simulink model "SF007A_SysFricLrng"  (R2013b)
settings: Solver=FixedStepDiscrete  SolverMode=SingleTasking  StartTime=0.0  StopTime=1  FixedStep=0.002  RelTol=1e-3
PostLoadFcn:
  | , if any(exist('dsrtsu_mdlpostloadfcn', 'file') == [2, 3, 6]), try dsrtsu_mdlpostloadfcn('Execute', bdroot); catch fprintf('Error in PostLoadFcn (dsrtsu_mdlpostloadfcn) for model "%s":\n %s\n', bdroot, lasterr); end, end,
values from neighbouring files (symbols this model uses):
  ARCHGLBPRM_100MILLISEC_SEC_F32 = DataDict.Constant    [SF007A_SysFricLrng_DataDict.m]
  ARCHGLBPRM_10MILLISEC_SEC_F32 = DataDict.Constant    [SF007A_SysFricLrng_DataDict.m]
  ARCHGLBPRM_180OVERPI_ULS_F32 = DataDict.Constant    [SF007A_SysFricLrng_DataDict.m]
  CONV100MICROSECTOSEC_ULS_F32 = DataDict.Constant    [SF007A_SysFricLrng_DataDict.m]
  FLTINJ_SYSFRICLRNG_SYSFRICOFFS = DataDict.Constant    [SF007A_SysFricLrng_DataDict.m]
  FricLrngData = DataDict.NVM    [SF007A_SysFricLrng_DataDict.m]
  HWPTNUM_CNT_U08 = DataDict.Constant    [SF007A_SysFricLrng_DataDict.m]
  HWPTNUMSUB1_CNT_U08 = DataDict.Constant    [SF007A_SysFricLrng_DataDict.m]
  HWVELDECDIR_ULS_U08 = DataDict.Constant    [SF007A_SysFricLrng_DataDict.m]
  HWVELINCDIR_ULS_U08 = DataDict.Constant    [SF007A_SysFricLrng_DataDict.m]
  IDXCALCNSCAGFAC_ULS_U08 = DataDict.Constant    [SF007A_SysFricLrng_DataDict.m]
  IDXSELN1_ULS_U08 = DataDict.Constant    [SF007A_SysFricLrng_DataDict.m]
  IDXSELN2_ULS_U08 = DataDict.Constant    [SF007A_SysFricLrng_DataDict.m]
  IDXSELN3_ULS_U08 = DataDict.Constant    [SF007A_SysFricLrng_DataDict.m]
  LRNGENASCAFAC_MILLISEC_U32 = DataDict.Constant    [SF007A_SysFricLrng_DataDict.m]
  SCAGFACQUARTER_CNT_F32 = DataDict.Constant    [SF007A_SysFricLrng_DataDict.m]
  SCAGFACTEN_CNT_U16 = DataDict.Constant    [SF007A_SysFricLrng_DataDict.m]
  SCAGFACVEHLATA_MTRPERSECSQD_F32 = DataDict.Constant    [SF007A_SysFricLrng_DataDict.m]
  SECIDXSELN_ULS_U08 = DataDict.Constant    [SF007A_SysFricLrng_DataDict.m]
  SysFricLrngBasLineEolFric = DataDict.Calibration    [SF007A_SysFricLrng_DataDict.m]
  SysFricLrngBasLineFric = DataDict.Calibration    [SF007A_SysFricLrng_DataDict.m]
  SysFricLrngBasLineHys = DataDict.Calibration    [SF007A_SysFricLrng_DataDict.m]
  SysFricLrngBasLineRngCntr = DataDict.Calibration    [SF007A_SysFricLrng_DataDict.m]
  SysFricLrngEolFricDifScagFac = DataDict.Calibration    [SF007A_SysFricLrng_DataDict.m]
  SysFricLrngFricChgWght = DataDict.Calibration    [SF007A_SysFricLrng_DataDict.m]
  SysFricLrngFricDiagcThd = DataDict.Calibration    [SF007A_SysFricLrng_DataDict.m]
  SysFricLrngFricDiagcTiThd = DataDict.Calibration    [SF007A_SysFricLrng_DataDict.m]
  SysFricLrngFricHysHwAgPt = DataDict.Calibration    [SF007A_SysFricLrng_DataDict.m]
  SysFricLrngGain = DataDict.Calibration    [SF007A_SysFricLrng_DataDict.m]
  SysFricLrngHwPosnAuthyThd = DataDict.Calibration    [SF007A_SysFricLrng_DataDict.m]
  SysFricLrngHwVelConstrLim = DataDict.Calibration    [SF007A_SysFricLrng_DataDict.m]
  SysFricLrngHwVelHiLim = DataDict.Calibration    [SF007A_SysFricLrng_DataDict.m]
  SysFricLrngHwVelLoLim = DataDict.Calibration    [SF007A_SysFricLrng_DataDict.m]
  SysFricLrngIgnCycFricChgLim = DataDict.Calibration    [SF007A_SysFricLrng_DataDict.m]
  SysFricLrngLatAHiLim = DataDict.Calibration    [SF007A_SysFricLrng_DataDict.m]
  SysFricLrngLatALoLim = DataDict.Calibration    [SF007A_SysFricLrng_DataDict.m]
  SysFricLrngMaskVehSpd = DataDict.Calibration    [SF007A_SysFricLrng_DataDict.m]
  SysFricLrngRngCntrThd = DataDict.Calibration    [SF007A_SysFricLrng_DataDict.m]
  SysFricLrngThd = DataDict.Calibration    [SF007A_SysFricLrng_DataDict.m]
  SysFricLrngTHiLim = DataDict.Calibration    [SF007A_SysFricLrng_DataDict.m]
  SysFricLrngTLoLim = DataDict.Calibration    [SF007A_SysFricLrng_DataDict.m]
  SysFricLrngVehSpd = DataDict.Calibration    [SF007A_SysFricLrng_DataDict.m]
  SYSFRICOFFSLIM_HWNWTMTR_F32 = DataDict.Constant    [SF007A_SysFricLrng_DataDict.m]
  VEHSPDPTNUM1_ULS_U08 = DataDict.Constant    [SF007A_SysFricLrng_DataDict.m]
  VEHSPDPTNUM2_ULS_U08 = DataDict.Constant    [SF007A_SysFricLrng_DataDict.m]
undefined symbols (not defined in the file or in its folder): NtcNr1, NtcSts1, SysFricLrngOperMod1
libraries: Fil x19, simulink x17, NxtrLim x10, NxtrAbslt x3, NxtrNvM x2, FixdToFloat x2, FloatToFixd x1, LnrIntrpn x1
(part 3 of 7)

== system SF007A_SysFricLrng/SysFricLrng/SysFricLrngPer1/RunningAndCalibrationModes/CalMode ==
  Action Port : ActionPort  ActionType=then
  Constant1 : Constant  Value=0  OutDataTypeStr=single
      settings: AttributesFormatString=%<OutDataTypeStr>
  Constant2 : Constant  Value=0  OutDataTypeStr=single
      settings: AttributesFormatString=%<OutDataTypeStr>
  CopyRight2 : Subsystem  Description=|  mask(Copyright Information){none=on}
      | Copyright info block.                                               
      |                                                                     
      | Place copyright information at the top of every subsystem in design.
      mask prompts: none "No parameters"
      mask help: Place copyright information at the top of every subsystem in design.
      mask Display:
      | NxtrConf = 'Nexteer Confidential';
      | 
      | sys = bdroot; %handle for the current model ("system")
      | first = get_param(sys,'Created');
      | first = first(end-3:end);  %year is last four digits
      | 
      | last = get_param(sys,'LastModifiedDate');
      | if isempty(last)
      |     last = datestr(now,'yyyy');
      | else
      |     last = last(end-3:end);
      | end
      | 
      | if strcmp(first,last)
      |     fprintf('%s -- Copyright %s Nexteer',NxtrConf,first)
      | else
      |     fprintf('%s -- %s%s- %s Nexteer',NxtrConf,char(169),first,last)
      | end
  Data Store Read3 : DataStoreRead  DataStoreName=SatnAvrgFric
  Data Store Write : DataStoreWrite  DataStoreName=VehBasLineFric
  Data Store Write1 : DataStoreWrite  DataStoreName=FricChgLpFil  DataStoreElements=FricChgLpFil.FilSt
  FricOffs : Outport  InitialOutput=[0]
  wires:
  Data Store Read3/1 -> Data Store Write/1
  Constant1/1 -> FricOffs/1
  Constant2/1 -> Data Store Write1/1

== system SF007A_SysFricLrng/SysFricLrng/SysFricLrngPer1/RunningAndCalibrationModes/CopyRight2 ==

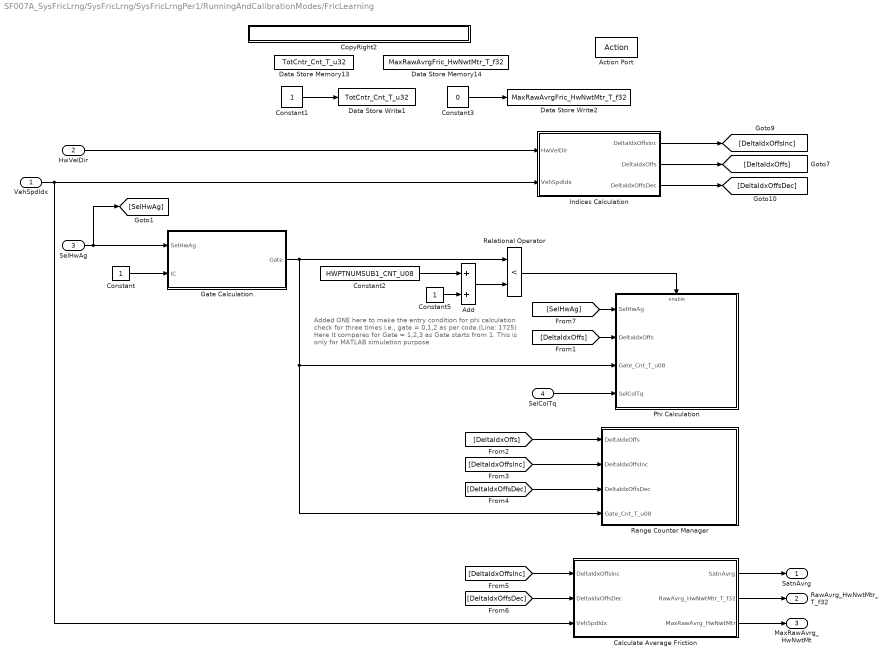
== system SF007A_SysFricLrng/SysFricLrng/SysFricLrngPer1/RunningAndCalibrationModes/FricLearning ==
  note: Added ONE here to make the entry condition for phi calculation
      | check for three times i.e., gate = 0,1,2 as per code.(Line: 1725)
      | Here It compares for Gate = 1,2,3 as Gate starts from 1.
      | This is only for MATLAB simulation purpose
  VehSpdIdx : Inport
  HwVelDir : Inport  Port=2
  SelHwAg : Inport  Port=3
  SelColTq : Inport  Port=4
  Action Port : ActionPort  ActionType=then
  Add : Sum
  Calculate Average Friction : Subsystem
  Constant : Constant  OutDataTypeStr=uint8
      settings: AttributesFormatString=%<OutDataTypeStr>
  Constant1 : Constant  OutDataTypeStr=uint32
      settings: AttributesFormatString=%<OutDataTypeStr>
  Constant2 : Constant  Value=HWPTNUMSUB1_CNT_U08
  Constant3 : Constant  Value=0  OutDataTypeStr=single
      settings: AttributesFormatString=%<OutDataTypeStr>
  Constant5 : Constant  OutDataTypeStr=uint16
      settings: AttributesFormatString=%<OutDataTypeStr>
  CopyRight2 : Subsystem  Description=|  mask(Copyright Information){none=on}
      | Copyright info block.                                               
      |                                                                     
      | Place copyright information at the top of every subsystem in design.
      mask prompts: none "No parameters"
      mask help: Place copyright information at the top of every subsystem in design.
      mask Display:
      | NxtrConf = 'Nexteer Confidential';
      | 
      | sys = bdroot; %handle for the current model ("system")
      | first = get_param(sys,'Created');
      | first = first(end-3:end);  %year is last four digits
      | 
      | last = get_param(sys,'LastModifiedDate');
      | if isempty(last)
      |     last = datestr(now,'yyyy');
      | else
      |     last = last(end-3:end);
      | end
      | 
      | if strcmp(first,last)
      |     fprintf('%s -- Copyright %s Nexteer',NxtrConf,first)
      | else
      |     fprintf('%s -- %s%s- %s Nexteer',NxtrConf,char(169),first,last)
      | end
  Data Store Memory13 : DataStoreMemory  Description=Local Data Store Memory  DataStoreName=TotCntr_Cnt_T_u32  OutDataTypeStr=uint32
      settings: AttributesFormatString=%<Description>
  Data Store Memory14 : DataStoreMemory  Description=Local Data Store Memory  DataStoreName=MaxRawAvrgFric_HwNwtMtr_T_f32  ReadBeforeWriteMsg=warning  WriteAfterWriteMsg=warning  WriteAfterReadMsg=warning  OutDataTypeStr=single
      settings: AttributesFormatString=%<Description>
  Data Store Write1 : DataStoreWrite  Priority=1  DataStoreName=TotCntr_Cnt_T_u32
      settings: AttributesFormatString=Priority:%<Priority>
  Data Store Write2 : DataStoreWrite  Priority=1  DataStoreName=MaxRawAvrgFric_HwNwtMtr_T_f32
      settings: AttributesFormatString=Priority:%<Priority>
  Gate Calculation : Subsystem  Priority=1  TreatAsAtomicUnit=on
      settings: AttributesFormatString=Priority:%<Priority>
  Indices Calculation : Subsystem
  Phi Calculation : Subsystem
  Range Counter Manager : Subsystem
  Relational Operator : RelationalOperator  Operator=<  OutDataTypeStr=boolean
  SatnAvrg : Outport
  RawAvrg_HwNwtMtr_T_f32 : Outport  Port=2
  MaxRawAvrg_HwNwtMt : Outport  Port=3
  wires:
  Constant1/1 -> Data Store Write1/1
  Constant3/1 -> Data Store Write2/1
  HwVelDir/1 -> Indices Calculation/1(HwVelDir)
  VehSpdIdx/1 -> Indices Calculation/2(VehSpdIdx), Calculate Average Friction/3(VehSpdIdx)
  Indices Calculation/1(DeltaIdxOffsInc) -> [DeltaIdxOffsInc]
  Indices Calculation/2(DeltaIdxOffs) -> [DeltaIdxOffs]
  Indices Calculation/3(DeltaIdxOffsDec) -> [DeltaIdxOffsDec]
  Constant/1 -> Gate Calculation/2(IC)
  Relational Operator/1 -> Phi Calculation/Enable
  SelHwAg/1 -> Gate Calculation/1(SelHwAg), [SelHwAg]
  [DeltaIdxOffs] -> Phi Calculation/2(DeltaIdxOffs)
  [DeltaIdxOffs] -> Range Counter Manager/1("DeltaIdxOffs ")
  [DeltaIdxOffsDec] -> Range Counter Manager/3(DeltaIdxOffsDec)
  [DeltaIdxOffsInc] -> Range Counter Manager/2(DeltaIdxOffsInc)
  [DeltaIdxOffsInc] -> Calculate Average Friction/1(DeltaIdxOffsInc)
  [DeltaIdxOffsDec] -> Calculate Average Friction/2(DeltaIdxOffsDec)
  Calculate Average Friction/1(SatnAvrg) -> SatnAvrg/1
  Calculate Average Friction/2(RawAvrg_HwNwtMtr_T_f32) -> RawAvrg_HwNwtMtr_T_f32/1
  [SelHwAg] -> Phi Calculation/1(SelHwAg)
  SelColTq/1 -> Phi Calculation/4(SelColTq)
  Gate Calculation/1(Gate) -> Phi Calculation/3(Gate_Cnt_T_u08), Range Counter Manager/4(Gate_Cnt_T_u08), Relational Operator/1
  Constant5/1 -> Add/2
  Add/1 -> Relational Operator/2
  Constant2/1 -> Add/1
  Calculate Average Friction/3(MaxRawAvrg_HwNwtMtr) -> MaxRawAvrg_HwNwtMt/1

== system SF007A_SysFricLrng/SysFricLrng/SysFricLrngPer1/RunningAndCalibrationModes/Hold Last value ==
  SatEstimdFric : Inport
  EstimdFric : Inport  Port=2
  MaxRawAvgFric : Inport  Port=3
  Action Port : ActionPort  ActionType=else
  CopyRight2 : Subsystem  Description=|  mask(Copyright Information){none=on}
      | Copyright info block.                                               
      |                                                                     
      | Place copyright information at the top of every subsystem in design.
      mask prompts: none "No parameters"
      mask help: Place copyright information at the top of every subsystem in design.
      mask Display:
      | NxtrConf = 'Nexteer Confidential';
      | 
      | sys = bdroot; %handle for the current model ("system")
      | first = get_param(sys,'Created');
      | first = first(end-3:end);  %year is last four digits
      | 
      | last = get_param(sys,'LastModifiedDate');
      | if isempty(last)
      |     last = datestr(now,'yyyy');
      | else
      |     last = last(end-3:end);
      | end
      | 
      | if strcmp(first,last)
      |     fprintf('%s -- Copyright %s Nexteer',NxtrConf,first)
      | else
      |     fprintf('%s -- %s%s- %s Nexteer',NxtrConf,char(169),first,last)
      | end
  SatEstimdFric_HwNwtMt1 : Outport
  EstimdFric_HwNwtMt2 : Outport  Port=2
  MaxRawAvrg_HwNwtMt : Outport  Port=3
  wires:
  MaxRawAvgFric/1 -> MaxRawAvrg_HwNwtMt/1
  EstimdFric/1 -> EstimdFric_HwNwtMt2/1
  SatEstimdFric/1 -> SatEstimdFric_HwNwtMt1/1

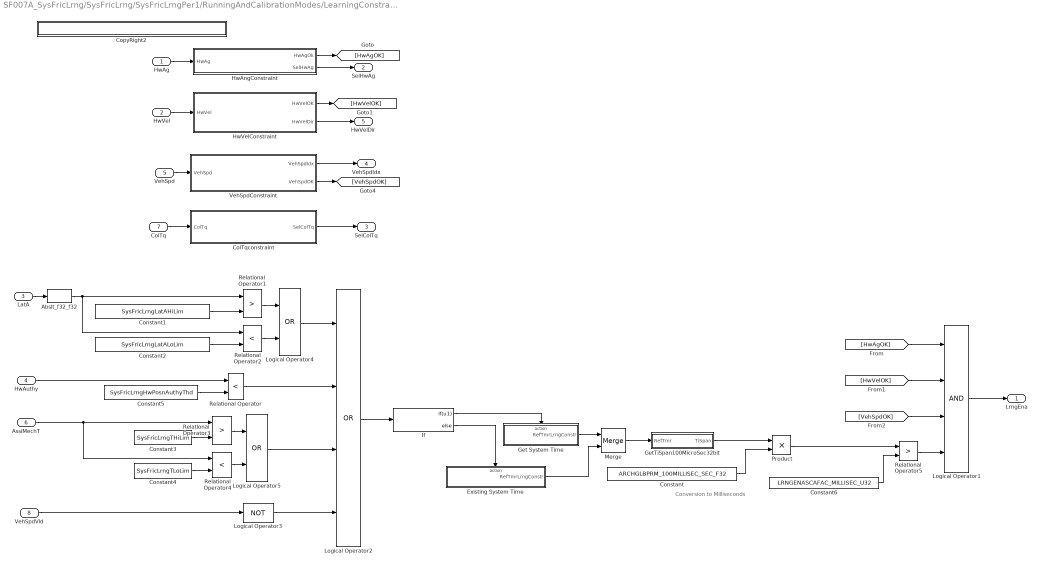
== system SF007A_SysFricLrng/SysFricLrng/SysFricLrngPer1/RunningAndCalibrationModes/LearningConstraint ==
  note: Conversion to Milliseconds
  HwAg : Inport
  HwVel : Inport  Port=2
  LatA : Inport  Port=3
  HwAuthy : Inport  Port=4
  VehSpd : Inport  Port=5
  AssiMechT : Inport  Port=6
  ColTq : Inport  Port=7
  VehSpdVld : Inport  Port=8
  Abslt_f32_f32 : NxtrAbslt/Abslt_f32_f32  SFunctionSpec=single y1 = Abslt_f32_f32(single u1)
      settings: AttributesFormatString=%<Name>
  ColTqconstraint : Subsystem
  Constant : Constant  Value=ARCHGLBPRM_100MILLISEC_SEC_F32
  Constant1 : Constant  Value=SysFricLrngLatAHiLim
  Constant2 : Constant  Value=SysFricLrngLatALoLim
  Constant3 : Constant  Value=SysFricLrngTHiLim
  Constant4 : Constant  Value=SysFricLrngTLoLim
  Constant5 : Constant  Value=SysFricLrngHwPosnAuthyThd
  Constant6 : Constant  Value=LRNGENASCAFAC_MILLISEC_U32
  CopyRight2 : Subsystem  Description=|  mask(Copyright Information){none=on}
      | Copyright info block.                                               
      |                                                                     
      | Place copyright information at the top of every subsystem in design.
      mask prompts: none "No parameters"
      mask help: Place copyright information at the top of every subsystem in design.
      mask Display:
      | NxtrConf = 'Nexteer Confidential';
      | 
      | sys = bdroot; %handle for the current model ("system")
      | first = get_param(sys,'Created');
      | first = first(end-3:end);  %year is last four digits
      | 
      | last = get_param(sys,'LastModifiedDate');
      | if isempty(last)
      |     last = datestr(now,'yyyy');
      | else
      |     last = last(end-3:end);
      | end
      | 
      | if strcmp(first,last)
      |     fprintf('%s -- Copyright %s Nexteer',NxtrConf,first)
      | else
      |     fprintf('%s -- %s%s- %s Nexteer',NxtrConf,char(169),first,last)
      | end
  Existing System Time : Subsystem  TreatAsAtomicUnit=on
  Get System Time : Subsystem  TreatAsAtomicUnit=on
  GetTiSpan100MicroSec32bit : Subsystem
  HwAngConstraint : Subsystem
  HwVelConstraint : Subsystem
  If : If  IfExpression=u1
  Logical Operator1 : Logic  Inputs=4  AllPortsSameDT=off  OutDataTypeStr=boolean
  Logical Operator2 : Logic  Operator=OR  Inputs=4  AllPortsSameDT=off  OutDataTypeStr=boolean
  Logical Operator3 : Logic  Operator=NOT  Inputs=4  AllPortsSameDT=off  OutDataTypeStr=boolean
  Logical Operator4 : Logic  Operator=OR  AllPortsSameDT=off  OutDataTypeStr=boolean
  Logical Operator5 : Logic  Operator=OR  AllPortsSameDT=off  OutDataTypeStr=boolean
  Merge : Merge
  Product : Product
  Relational Operator : RelationalOperator  Operator=<  OutDataTypeStr=boolean
  Relational Operator1 : RelationalOperator  Operator=>  OutDataTypeStr=boolean
  Relational Operator2 : RelationalOperator  Operator=<  OutDataTypeStr=boolean
  Relational Operator3 : RelationalOperator  Operator=>  OutDataTypeStr=boolean
  Relational Operator4 : RelationalOperator  Operator=<  OutDataTypeStr=boolean
  Relational Operator5 : RelationalOperator  Operator=>  OutDataTypeStr=boolean
  VehSpdConstraint : Subsystem
  LrngEna : Outport
  SelHwAg : Outport  Port=2
  SelColTq : Outport  Port=3
  VehSpdIdx : Outport  Port=4
  HwVelDir : Outport  Port=5
  wires:
  HwAg/1 -> HwAngConstraint/1(HwAg)
  HwVel/1 -> HwVelConstraint/1(HwVel)
  Logical Operator1/1 -> LrngEna/1
  VehSpd/1 -> VehSpdConstraint/1(VehSpd)
  HwAngConstraint/1(HwAgOk) -> [HwAgOK]
  ColTq/1 -> ColTqconstraint/1(ColTq)
  ColTqconstraint/1(SelColTq) -> SelColTq/1
  HwAngConstraint/2(SelHwAg) -> SelHwAg/1
  [HwAgOK] -> Logical Operator1/1
  [HwVelOK] -> Logical Operator1/2
  [VehSpdOK] -> Logical Operator1/3
  HwVelConstraint/2(HwVelDir) -> HwVelDir/1
  HwVelConstraint/1(HwVelOK) -> [HwVelOK]
  LatA/1 -> Abslt_f32_f32/1
  Abslt_f32_f32/1 -> Relational Operator1/1, Relational Operator2/1
  HwAuthy/1 -> Relational Operator/1
  Constant5/1 -> Relational Operator/2
  Relational Operator/1 -> Logical Operator2/2
  AssiMechT/1 -> Relational Operator3/1, Relational Operator4/1
  VehSpdConstraint/1(VehSpdIdx) -> VehSpdIdx/1
  VehSpdConstraint/2(VehSpdOK) -> [VehSpdOK]
  Relational Operator5/1 -> Logical Operator1/4
  Constant/1 -> Product/2
  Merge/1 -> GetTiSpan100MicroSec32bit/1(RefTmr)
  Get System Time/1(RefTmrLrngConstr) -> Merge/1
  Existing System Time/1(RefTmrLrngConstr) -> Merge/2
  If/1 -> Get System Time/Action
  If/2 -> Existing System Time/Action
  GetTiSpan100MicroSec32bit/1(TiSpan) -> Product/1
  Logical Operator4/1 -> Logical Operator2/1
  Logical Operator5/1 -> Logical Operator2/3
  VehSpdVld/1 -> Logical Operator3/1
  Constant1/1 -> Relational Operator1/2
  Relational Operator2/1 -> Logical Operator4/2
  Relational Operator1/1 -> Logical Operator4/1
  Constant2/1 -> Relational Operator2/2
  Constant3/1 -> Relational Operator3/2
  Constant4/1 -> Relational Operator4/2
  Relational Operator3/1 -> Logical Operator5/1
  Relational Operator4/1 -> Logical Operator5/2
  Logical Operator3/1 -> Logical Operator2/4
  Logical Operator2/1 -> If/1
  Product/1 -> Relational Operator5/1
  Constant6/1 -> Relational Operator5/2

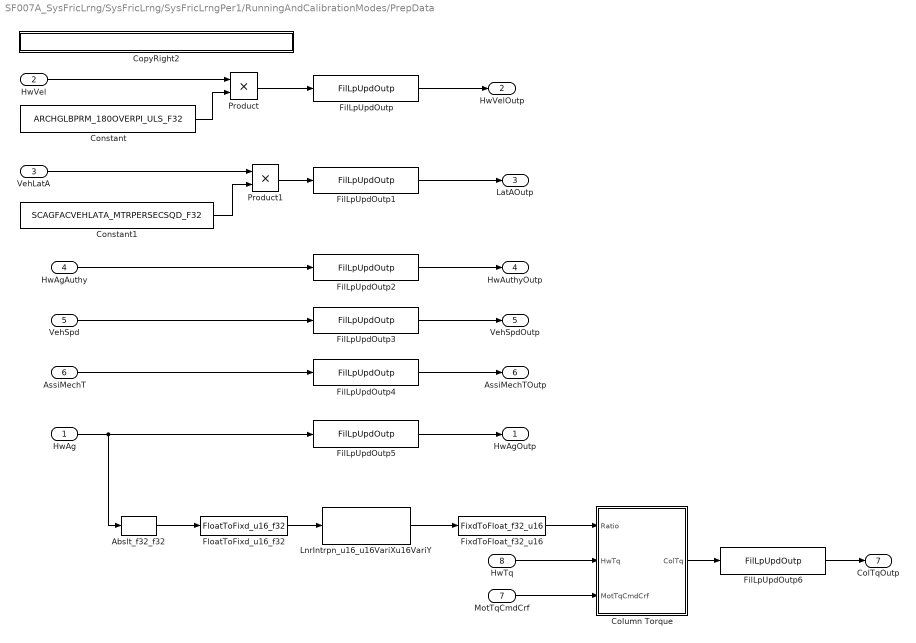
== system SF007A_SysFricLrng/SysFricLrng/SysFricLrngPer1/RunningAndCalibrationModes/PrepData ==
  HwAg : Inport
  HwVel : Inport  Port=2
  VehLatA : Inport  Port=3
  HwAgAuthy : Inport  Port=4
  VehSpd : Inport  Port=5
  AssiMechT : Inport  Port=6
  MotTqCmdCrf : Inport  Port=7
  HwTq : Inport  Port=8
  Abslt_f32_f32 : NxtrAbslt/Abslt_f32_f32  SFunctionSpec=single y1 = Abslt_f32_f32(single u1)
      settings: AttributesFormatString=%<Name>
  Column Torque : Subsystem
  Constant : Constant  Value=ARCHGLBPRM_180OVERPI_ULS_F32
  Constant1 : Constant  Value=SCAGFACVEHLATA_MTRPERSECSQD_F32
  CopyRight2 : Subsystem  Description=|  mask(Copyright Information){none=on}
      | Copyright info block.                                               
      |                                                                     
      | Place copyright information at the top of every subsystem in design.
      mask prompts: none "No parameters"
      mask help: Place copyright information at the top of every subsystem in design.
      mask Display:
      | NxtrConf = 'Nexteer Confidential';
      | 
      | sys = bdroot; %handle for the current model ("system")
      | first = get_param(sys,'Created');
      | first = first(end-3:end);  %year is last four digits
      | 
      | last = get_param(sys,'LastModifiedDate');
      | if isempty(last)
      |     last = datestr(now,'yyyy');
      | else
      |     last = last(end-3:end);
      | end
      | 
      | if strcmp(first,last)
      |     fprintf('%s -- Copyright %s Nexteer',NxtrConf,first)
      | else
      |     fprintf('%s -- %s%s- %s Nexteer',NxtrConf,char(169),first,last)
      | end
  FilLpUpdOutp : Fil/FilLpUpdOutp  StVar=HwVelLpFil
      settings: AttributesFormatString=StVar: %<StVar>
  FilLpUpdOutp1 : Fil/FilLpUpdOutp  StVar=LatALpFil
      settings: AttributesFormatString=StVar: %<StVar>
  FilLpUpdOutp2 : Fil/FilLpUpdOutp  StVar=HwAgAuthyLpFil
      settings: AttributesFormatString=StVar: %<StVar>
  FilLpUpdOutp3 : Fil/FilLpUpdOutp  StVar=VehSpdLpFil
      settings: AttributesFormatString=StVar: %<StVar>
  FilLpUpdOutp4 : Fil/FilLpUpdOutp  StVar=AssiMechTLpFil
      settings: AttributesFormatString=StVar: %<StVar>
  FilLpUpdOutp5 : Fil/FilLpUpdOutp  StVar=HwAgLpFil
      settings: AttributesFormatString=StVar: %<StVar>
  FilLpUpdOutp6 : Fil/FilLpUpdOutp  StVar=ColTqLpFil
      settings: AttributesFormatString=StVar: %<StVar>
  FixdToFloat_f32_u16 : FixdToFloat/FixdToFloat_f32_u16  Param1=10
  FloatToFixd_u16_f32 : FloatToFixd/FloatToFixd_u16_f32  Param1=5
  LnrIntrpn_u16_u16VariXu16VariY : LnrIntrpn/LnrIntrpn_u16_u16VariXu16VariY  XTbl=SysFricLrngIvsTrsmRatX  YTbl=SysFricLrngIvsTrsmRatY
      settings: AttributesFormatString=Lnr ( u16VariX , u16VariY )
  Product : Product
  Product1 : Product
  HwAgOutp : Outport
  HwVelOutp : Outport  Port=2
  LatAOutp : Outport  Port=3
  HwAuthyOutp : Outport  Port=4
  VehSpdOutp : Outport  Port=5
  AssiMechTOutp : Outport  Port=6
  ColTqOutp : Outport  Port=7
  wires:
  HwAg/1 -> Abslt_f32_f32/1, FilLpUpdOutp5/1
  HwVel/1 -> Product/1
  HwAgAuthy/1 -> FilLpUpdOutp2/1
  VehSpd/1 -> FilLpUpdOutp3/1
  AssiMechT/1 -> FilLpUpdOutp4/1
  FixdToFloat_f32_u16/1 -> Column Torque/1(Ratio)
  MotTqCmdCrf/1 -> Column Torque/3(MotTqCmdCrf)
  HwTq/1 -> Column Torque/2(HwTq)
  Column Torque/1(ColTq) -> FilLpUpdOutp6/1
  FilLpUpdOutp6/1 -> ColTqOutp/1
  FilLpUpdOutp/1 -> HwVelOutp/1
  FilLpUpdOutp1/1 -> LatAOutp/1
  FilLpUpdOutp2/1 -> HwAuthyOutp/1
  FilLpUpdOutp5/1 -> HwAgOutp/1
  FilLpUpdOutp3/1 -> VehSpdOutp/1
  FilLpUpdOutp4/1 -> AssiMechTOutp/1
  Abslt_f32_f32/1 -> FloatToFixd_u16_f32/1
  Product/1 -> FilLpUpdOutp/1
  FloatToFixd_u16_f32/1 -> LnrIntrpn_u16_u16VariXu16VariY/1
  LnrIntrpn_u16_u16VariXu16VariY/1 -> FixdToFloat_f32_u16/1
  Constant/1 -> Product/2
  VehLatA/1 -> Product1/1
  Product1/1 -> FilLpUpdOutp1/1
  Constant1/1 -> Product1/2

== system SF007A_SysFricLrng/SysFricLrng/SysFricLrngPer1/RunningAndCalibrationModes/Running Mode ==
  note: Input Portsize for the selector is size(SysFricLrngVehSpd,1)
  LrngEna : Inport
  VehSpdIdx : Inport  Port=2
  Action Port : ActionPort  ActionType=else
  CopyRight2 : Subsystem  Description=|  mask(Copyright Information){none=on}
      | Copyright info block.                                               
      |                                                                     
      | Place copyright information at the top of every subsystem in design.
      mask prompts: none "No parameters"
      mask help: Place copyright information at the top of every subsystem in design.
      mask Display:
      | NxtrConf = 'Nexteer Confidential';
      | 
      | sys = bdroot; %handle for the current model ("system")
      | first = get_param(sys,'Created');
      | first = first(end-3:end);  %year is last four digits
      | 
      | last = get_param(sys,'LastModifiedDate');
      | if isempty(last)
      |     last = datestr(now,'yyyy');
      | else
      |     last = last(end-3:end);
      | end
      | 
      | if strcmp(first,last)
      |     fprintf('%s -- Copyright %s Nexteer',NxtrConf,first)
      | else
      |     fprintf('%s -- %s%s- %s Nexteer',NxtrConf,char(169),first,last)
      | end
  Data Store Read : DataStoreRead  Priority=1  DataStoreName=PrevFricOffs
      settings: AttributesFormatString=Priority=%<Priority>
  Data Store Write : DataStoreWrite  Priority=2  DataStoreName=PrevFricOffs
      settings: AttributesFormatString=Priority=%<Priority>
  Else Action : Subsystem  TreatAsAtomicUnit=on
  If : If  IfExpression=u1
  If Action Subsystem : Subsystem  TreatAsAtomicUnit=on
  Merge : Merge
  FricOffs : Outport
  wires:
  LrngEna/1 -> If/1
  If/1 -> If Action Subsystem/Action
  VehSpdIdx/1 -> If Action Subsystem/1(VehSpdIdx)
  If Action Subsystem/1(FricOffs) -> Merge/1
  If/2 -> Else Action/Action
  Data Store Read/1 -> Else Action/1(In1)
  Else Action/1(Out1) -> Merge/2
  Merge/1 -> Data Store Write/1, FricOffs/1

== system SF007A_SysFricLrng/SysFricLrng/SysFricLrngPer1/UpdateNvmPrm/UpdateVehLearnedFric ==
  note: The magnitude of change is limited per a calibration value.
  ItrnLim : Inport
  Add2 : Sum
  Add3 : Sum  Inputs=+-
  Assignment : Assignment  RequirementInfo={} %GIDa_6b461834_d19c_44da_acbb_89104afb76e3  IndexOptions=Index vector (port)  Indices=1  OutputSizes=1
  Constant3 : Constant  Value=SysFricLrngIgnCycFricChgLim
  Constant4 : Constant  Value=SysFricLrngIgnCycFricChgLim
  Data Store Read : DataStoreRead  DataStoreName=FricLrngData  DataStoreElements=FricLrngData.VehLrndFric(:,:)
  Data Store Read1 : DataStoreRead  DataStoreName=FricLrngData  DataStoreElements=FricLrngData.VehLrndFric(:,:)
  Data Store Read6 : DataStoreRead  DataStoreName=SatnAvrgFric
  Data Store Write : DataStoreWrite  DataStoreName=FricLrngData  DataStoreElements=FricLrngData.VehLrndFric(:,:)
  For Iterator : ForIterator  IterationSource=external
  LimDyn_f32 : NxtrLim/LimDyn_f32
  LimStat_f4 : NxtrLim/LimStat_f32  LoLim=VEHLRNDFRICLOLIM_ULS_F32  HiLim=VEHLRNDFRICHILIM_ULS_F32
      settings: AttributesFormatString=|
      | Low Limit: %<LoLim>
      | High Limit:%<HiLim>
  Selector1 : Selector  InputPortWidth=4  IndexOptions=Index vector (port)  Indices=[1 3]  OutputSizes=1
  Selector2 : Selector  InputPortWidth=4  IndexOptions=Index vector (port)  Indices=[1 3]  OutputSizes=1
  wires:
  ItrnLim/1 -> For Iterator/1
  For Iterator/1 -> Assignment/3, Selector1/2, Selector2/2
  Data Store Read6/1 -> Selector2/1
  Data Store Read/1 -> Selector1/1
  Assignment/1 -> Data Store Write/1
  Data Store Read1/1 -> Assignment/1
  Constant3/1 -> Add2/2
  Selector1/1 -> Add2/1, Add3/2
  Constant4/1 -> Add3/1
  LimStat_f4/1 -> Assignment/2
  LimDyn_f32/1 -> LimStat_f4/1
  Selector2/1 -> LimDyn_f32/1
  Add2/1 -> LimDyn_f32/3
  Add3/1 -> LimDyn_f32/2

== system SF007A_SysFricLrng/SysFricLrng/SysFricLrngPer1/enable/CopyRight2 ==

== system SF007A_SysFricLrng/SysFricLrng/SysFricLrngPer1/updateNvmOperMode/CopyRight2 ==

== system SF007A_SysFricLrng/SysFricLrng/SysFricLrngInit1/Initialization/InitAvrgFricLpFil1/CopyRight2 ==

== system SF007A_SysFricLrng/SysFricLrng/SysFricLrngInit1/Initialization/InitAvrgFricLpFil2/CopyRight2 ==

== system SF007A_SysFricLrng/SysFricLrng/SysFricLrngInit1/Initialization/InitAvrgFricLpFil3/CopyRight2 ==

== system SF007A_SysFricLrng/SysFricLrng/SysFricLrngInit1/Initialization/InitAvrgFricLpFil4/CopyRight2 ==

== system SF007A_SysFricLrng/SysFricLrng/SysFricLrngPer1/ResettingMode (reset to baseline) (rename this mode as InitializeTable)/UpdateBaselineFric/CopyRight2 ==

== system SF007A_SysFricLrng/SysFricLrng/SysFricLrngPer1/ResettingMode (reset to baseline) (rename this mode as InitializeTable)/UpdateBaselineFric/InitAvrgFricLpFil1 ==
  LrndBaselineFric : Inport
  Action Port : ActionPort  ActionType=case
  CopyRight2 : Subsystem  Description=|  mask(Copyright Information){none=on}
      | Copyright info block.                                               
      |                                                                     
      | Place copyright information at the top of every subsystem in design.
      mask prompts: none "No parameters"
      mask help: Place copyright information at the top of every subsystem in design.
      mask Display:
      | NxtrConf = 'Nexteer Confidential';
      | 
      | sys = bdroot; %handle for the current model ("system")
      | first = get_param(sys,'Created');
      | first = first(end-3:end);  %year is last four digits
      | 
      | last = get_param(sys,'LastModifiedDate');
      | if isempty(last)
      |     last = datestr(now,'yyyy');
      | else
      |     last = last(end-3:end);
      | end
      | 
      | if strcmp(first,last)
      |     fprintf('%s -- Copyright %s Nexteer',NxtrConf,first)
      | else
      |     fprintf('%s -- %s%s- %s Nexteer',NxtrConf,char(169),first,last)
      | end
  Data Store Write : DataStoreWrite  DataStoreName=AvrgFricLpFil1  DataStoreElements=AvrgFricLpFil1.FilSt
  wires:
  LrndBaselineFric/1 -> Data Store Write/1

== system SF007A_SysFricLrng/SysFricLrng/SysFricLrngPer1/ResettingMode (reset to baseline) (rename this mode as InitializeTable)/UpdateBaselineFric/InitAvrgFricLpFil2 ==
  LrndBaselineFric : Inport
  Action Port : ActionPort  ActionType=case
  CopyRight2 : Subsystem  Description=|  mask(Copyright Information){none=on}
      | Copyright info block.                                               
      |                                                                     
      | Place copyright information at the top of every subsystem in design.
      mask prompts: none "No parameters"
      mask help: Place copyright information at the top of every subsystem in design.
      mask Display:
      | NxtrConf = 'Nexteer Confidential';
      | 
      | sys = bdroot; %handle for the current model ("system")
      | first = get_param(sys,'Created');
      | first = first(end-3:end);  %year is last four digits
      | 
      | last = get_param(sys,'LastModifiedDate');
      | if isempty(last)
      |     last = datestr(now,'yyyy');
      | else
      |     last = last(end-3:end);
      | end
      | 
      | if strcmp(first,last)
      |     fprintf('%s -- Copyright %s Nexteer',NxtrConf,first)
      | else
      |     fprintf('%s -- %s%s- %s Nexteer',NxtrConf,char(169),first,last)
      | end
  Data Store Write : DataStoreWrite  DataStoreName=AvrgFricLpFil2  DataStoreElements=AvrgFricLpFil2.FilSt
  wires:
  LrndBaselineFric/1 -> Data Store Write/1

== system SF007A_SysFricLrng/SysFricLrng/SysFricLrngPer1/ResettingMode (reset to baseline) (rename this mode as InitializeTable)/UpdateBaselineFric/InitAvrgFricLpFil3 ==
  LrndBaselineFric : Inport
  Action Port : ActionPort  ActionType=case
  CopyRight2 : Subsystem  Description=|  mask(Copyright Information){none=on}
      | Copyright info block.                                               
      |                                                                     
      | Place copyright information at the top of every subsystem in design.
      mask prompts: none "No parameters"
      mask help: Place copyright information at the top of every subsystem in design.
      mask Display:
      | NxtrConf = 'Nexteer Confidential';
      | 
      | sys = bdroot; %handle for the current model ("system")
      | first = get_param(sys,'Created');
      | first = first(end-3:end);  %year is last four digits
      | 
      | last = get_param(sys,'LastModifiedDate');
      | if isempty(last)
      |     last = datestr(now,'yyyy');
      | else
      |     last = last(end-3:end);
      | end
      | 
      | if strcmp(first,last)
      |     fprintf('%s -- Copyright %s Nexteer',NxtrConf,first)
      | else
      |     fprintf('%s -- %s%s- %s Nexteer',NxtrConf,char(169),first,last)
      | end
  Data Store Write : DataStoreWrite  DataStoreName=AvrgFricLpFil3  DataStoreElements=AvrgFricLpFil3.FilSt
  wires:
  LrndBaselineFric/1 -> Data Store Write/1

== system SF007A_SysFricLrng/SysFricLrng/SysFricLrngPer1/ResettingMode (reset to baseline) (rename this mode as InitializeTable)/UpdateBaselineFric/InitAvrgFricLpFil4 ==
  LrndBaselineFric : Inport
  Action Port : ActionPort  ActionType=default
  CopyRight2 : Subsystem  Description=|  mask(Copyright Information){none=on}
      | Copyright info block.                                               
      |                                                                     
      | Place copyright information at the top of every subsystem in design.
      mask prompts: none "No parameters"
      mask help: Place copyright information at the top of every subsystem in design.
      mask Display:
      | NxtrConf = 'Nexteer Confidential';
      | 
      | sys = bdroot; %handle for the current model ("system")
      | first = get_param(sys,'Created');
      | first = first(end-3:end);  %year is last four digits
      | 
      | last = get_param(sys,'LastModifiedDate');
      | if isempty(last)
      |     last = datestr(now,'yyyy');
      | else
      |     last = last(end-3:end);
      | end
      | 
      | if strcmp(first,last)
      |     fprintf('%s -- Copyright %s Nexteer',NxtrConf,first)
      | else
      |     fprintf('%s -- %s%s- %s Nexteer',NxtrConf,char(169),first,last)
      | end
  Data Store Write : DataStoreWrite  DataStoreName=AvrgFricLpFil4  DataStoreElements=AvrgFricLpFil4.FilSt
  wires:
  LrndBaselineFric/1 -> Data Store Write/1

== system SF007A_SysFricLrng/SysFricLrng/SysFricLrngPer1/ResettingMode (reset to baseline) (rename this mode as InitializeTable)/UpdateFricLrngHys_RngCntr/CopyRight2 ==

== system SF007A_SysFricLrng/SysFricLrng/SysFricLrngPer1/ResettingMode (reset to baseline) (rename this mode as InitializeTable)/UpdateFricLrngHys_RngCntr/Update BaseLine Range Counter ==
  note: Don't code this
  VehspdPtNumIdx : Inport
  HWPTNUMSUB1_CNT_U08 : Inport  Port=2
  Assignment1 : Assignment  NumberOfDimensions=2  IndexOptions=Index vector (port),Index vector (port)  Indices=1,1  OutputSizes=1,1
  Constant2 : Constant  Value=SysFricLrngBasLineRngCntr
  CopyRight2 : Subsystem  Description=|  mask(Copyright Information){none=on}
      | Copyright info block.                                               
      |                                                                     
      | Place copyright information at the top of every subsystem in design.
      mask prompts: none "No parameters"
      mask help: Place copyright information at the top of every subsystem in design.
      mask Display:
      | NxtrConf = 'Nexteer Confidential';
      | 
      | sys = bdroot; %handle for the current model ("system")
      | first = get_param(sys,'Created');
      | first = first(end-3:end);  %year is last four digits
      | 
      | last = get_param(sys,'LastModifiedDate');
      | if isempty(last)
      |     last = datestr(now,'yyyy');
      | else
      |     last = last(end-3:end);
      | end
      | 
      | if strcmp(first,last)
      |     fprintf('%s -- Copyright %s Nexteer',NxtrConf,first)
      | else
      |     fprintf('%s -- %s%s- %s Nexteer',NxtrConf,char(169),first,last)
      | end
  Data Store Read : DataStoreRead  Priority=1  DataStoreName=FricLrngData  DataStoreElements=FricLrngData.RngCntr(:,:)
      settings: AttributesFormatString=Priority:%<Priority>
  Data Store Write8 : DataStoreWrite  Priority=2  DataStoreName=FricLrngData  DataStoreElements=FricLrngData.RngCntr(:,:)
      settings: AttributesFormatString=Priority:%<Priority>
  Data Type Conversion : DataTypeConversion  OutDataTypeStr=uint8
  For Iterator : ForIterator  IterationSource=external  IterationVariableDataType=int16
  Selector1 : Selector  NumberOfDimensions=2  InputPortWidth=8  IndexOptions=Index vector (port),Index vector (port)  Indices=[1 3],1  OutputSizes=1,1
  Transpose1 : Math  Operator=transpose  SaturateOnIntegerOverflow=on
  wires:
  For Iterator/1 -> Data Type Conversion/1  "HwPtNumSub1"
  Data Store Read/1 -> Assignment1/1
  Assignment1/1 -> Data Store Write8/1
  Constant2/1 -> Transpose1/1
  Data Type Conversion/1 -> Assignment1/4, Selector1/3
  VehspdPtNumIdx/1 -> Selector1/2, Assignment1/3
  Selector1/1 -> Assignment1/2
  HWPTNUMSUB1_CNT_U08/1 -> For Iterator/1
  Transpose1/1 -> Selector1/1

== system SF007A_SysFricLrng/SysFricLrng/SysFricLrngPer1/ResettingMode (reset to baseline) (rename this mode as InitializeTable)/UpdateFricLrngHys_RngCntr/UpdateFricLrngHys ==
  HWPTNUM_CNT_U08 : Inport
  EolFricDif : Inport  Port=2
  VehspdPtNumIdx : Inport  Port=3
  Bitwise Operator : simulink/Logic and Bit Operations/Bitwise Operator  logicop=AND  UseBitMask=off  NumInputPorts=2  BitMask=bin2dec('11011001')  BitMaskRealWorld=Stored Integer
  Constant : Constant  OutDataTypeStr=uint8
      settings: AttributesFormatString=%<OutDataTypeStr>
  Constant1 : Constant  OutDataTypeStr=uint8
      settings: AttributesFormatString=%<OutDataTypeStr>
  CopyRight2 : Subsystem  Description=|  mask(Copyright Information){none=on}
      | Copyright info block.                                               
      |                                                                     
      | Place copyright information at the top of every subsystem in design.
      mask prompts: none "No parameters"
      mask help: Place copyright information at the top of every subsystem in design.
      mask Display:
      | NxtrConf = 'Nexteer Confidential';
      | 
      | sys = bdroot; %handle for the current model ("system")
      | first = get_param(sys,'Created');
      | first = first(end-3:end);  %year is last four digits
      | 
      | last = get_param(sys,'LastModifiedDate');
      | if isempty(last)
      |     last = datestr(now,'yyyy');
      | else
      |     last = last(end-3:end);
      | end
      | 
      | if strcmp(first,last)
      |     fprintf('%s -- Copyright %s Nexteer',NxtrConf,first)
      | else
      |     fprintf('%s -- %s%s- %s Nexteer',NxtrConf,char(169),first,last)
      | end
  Data Type Conversion : DataTypeConversion  OutDataTypeStr=uint8
  Even Rows : Subsystem  TreatAsAtomicUnit=on
  For Iterator : ForIterator  IterationSource=external  IterationVariableDataType=int16
  If : If  IfExpression=u1
  Odd Rows : Subsystem  TreatAsAtomicUnit=on
  Relational Operator : RelationalOperator  Operator===  OutDataTypeStr=boolean
  Subtract : Sum  Inputs=+-
  wires:
  For Iterator/1 -> Data Type Conversion/1
  Constant/1 -> Bitwise Operator/2, Relational Operator/2
  Bitwise Operator/1 -> Relational Operator/1
  Relational Operator/1 -> If/1
  If/1 -> Odd Rows/Action
  VehspdPtNumIdx/1 -> [VehspdPtNumIdx], Subtract/1
  [HwPtNumIdx] -> Odd Rows/1(HwPtNumIdx)
  [VehspdPtNumIdx] -> Odd Rows/2(VehspdPtNumIdx)
  [HwPtNumIdx] -> Even Rows/1(HwPtNumIdx)
  [VehspdPtNumIdx] -> Even Rows/2(VehspdPtNumIdx)
  If/2 -> Even Rows/Action
  EolFricDif/1 -> [EolFricDif]
  [EolFricDif] -> Odd Rows/3(EolFricDif)
  [EolFricDif] -> Even Rows/3(EolFricDif)
  Data Type Conversion/1 -> [HwPtNumIdx]
  HWPTNUM_CNT_U08/1 -> For Iterator/1
  Subtract/1 -> Bitwise Operator/1
  Constant1/1 -> Subtract/2

== system SF007A_SysFricLrng/SysFricLrng/SysFricLrngPer1/RunningAndCalibrationModes/CalMode/CopyRight2 ==

== system SF007A_SysFricLrng/SysFricLrng/SysFricLrngPer1/RunningAndCalibrationModes/FricLearning/Calculate Average Friction ==
  note: Abs block removed as value of 'MaxRawAvrgFric'
      |  will never be negative value
  DeltaIdxOffsInc : Inport
  DeltaIdxOffsDec : Inport  Port=2
  VehSpdIdx : Inport  Port=3
  Constant1 : Constant  Value=VEHSPDPTNUM1_ULS_U08
  Constant2 : Constant  Value=SysFricLrngThd
  Constant3 : Constant  OutDataTypeStr=uint8
      settings: AttributesFormatString=%<OutDataTypeStr>
  Constant4 : Constant  Value=SysFricLrngFricDiagcThd
  Constant5 : Constant  Value=HWPTNUMSUB1_CNT_U08
  Constant8 : Constant  Value=0  OutDataTypeStr=uint8
      settings: AttributesFormatString=%<OutDataTypeStr>
  CopyRight2 : Subsystem  Description=|  mask(Copyright Information){none=on}
      | Copyright info block.                                               
      |                                                                     
      | Place copyright information at the top of every subsystem in design.
      mask prompts: none "No parameters"
      mask help: Place copyright information at the top of every subsystem in design.
      mask Display:
      | NxtrConf = 'Nexteer Confidential';
      | 
      | sys = bdroot; %handle for the current model ("system")
      | first = get_param(sys,'Created');
      | first = first(end-3:end);  %year is last four digits
      | 
      | last = get_param(sys,'LastModifiedDate');
      | if isempty(last)
      |     last = datestr(now,'yyyy');
      | else
      |     last = last(end-3:end);
      | end
      | 
      | if strcmp(first,last)
      |     fprintf('%s -- Copyright %s Nexteer',NxtrConf,first)
      | else
      |     fprintf('%s -- %s%s- %s Nexteer',NxtrConf,char(169),first,last)
      | end
  Data Store Read1 : DataStoreRead  Priority=2  DataStoreName=MaxRawAvrgFric_HwNwtMtr_T_f32
      settings: AttributesFormatString=Priority: %<Priority>
  Data Store Read2 : DataStoreRead  Priority=2  DataStoreName=TotCntr_Cnt_T_u32
      settings: AttributesFormatString=Priority:%<Priority>
  Enumerated Constant1 : simulink/Sources/Enumerated Constant  OutDataTypeStr=Enum: NtcSts1  Value=NtcSts1.NTCSTS_FAILD  SampleTime=inf
  Enumerated Constant2 : simulink/Sources/Enumerated Constant  OutDataTypeStr=Enum: NtcSts1  Value=NtcSts1.NTCSTS_PASSD  SampleTime=inf
  Ground : Ground
  Ground1 : Ground
  HiFricNtc : simulink/Sources/Enumerated Constant  OutDataTypeStr=Enum: NtcNr1  Value=NtcNr1.NTCNR_0X0A2  SampleTime=inf
  HiFricNtc1 : simulink/Sources/Enumerated Constant  OutDataTypeStr=Enum: NtcNr1  Value=NtcNr1.NTCNR_0X0A2  SampleTime=inf
  If : If  IfExpression=u1
  Max Raw Average Calculation : Subsystem  Priority=1  TreatAsAtomicUnit=on
      settings: AttributesFormatString=Priority:%<Priority>
  NTC FAIL : Subsystem  TreatAsAtomicUnit=on
  "NTC PASS " : Subsystem  TreatAsAtomicUnit=on
  Raw Average Calculation : Subsystem  TreatAsAtomicUnit=on
  Relational Operator : RelationalOperator  OutDataTypeStr=boolean
  Relational Operator1 : RelationalOperator  OutDataTypeStr=boolean
  Total Counter Updation : Subsystem  Priority=1  TreatAsAtomicUnit=on
      settings: AttributesFormatString=Priority:%<Priority>
  SatnAvrg : Outport
  RawAvrg_HwNwtMtr_T_f32 : Outport  Port=2
  MaxRawAvrg_HwNwtMtr : Outport  Port=3
  wires:
  DeltaIdxOffsInc/1 -> Total Counter Updation/2(DeltaIdxOffsInc), Raw Average Calculation/2(DeltaIdxOffsInc)
  DeltaIdxOffsDec/1 -> Raw Average Calculation/1(DeltaIdxOffsDec), Total Counter Updation/3(DeltaIdxOffsDec)
  Data Store Read2/1 -> Relational Operator/1
  Constant2/1 -> Relational Operator/2
  Relational Operator/1 -> Raw Average Calculation/Enable
  VehSpdIdx/1 -> Raw Average Calculation/3(VehSpdIdx)
  Raw Average Calculation/1(SatnAvrg) -> SatnAvrg/1
  Raw Average Calculation/2(RawAvrg_HwNwtMtr_T_f32) -> RawAvrg_HwNwtMtr_T_f32/1
  If/1 -> NTC FAIL/Action
  If/2 -> "NTC PASS "/Action
  Relational Operator1/1 -> If/1
  Constant3/1 -> NTC FAIL/2(NtcStInfo)
  HiFricNtc/1 -> NTC FAIL/1(NtcNr)
  HiFricNtc1/1 -> "NTC PASS "/1(NtcNr)
  Constant8/1 -> "NTC PASS "/2(NtcStInfo)
  Enumerated Constant1/1 -> NTC FAIL/3(NtcSts)
  Ground/1 -> NTC FAIL/4(DebStep)
  Ground1/1 -> "NTC PASS "/4(DebStep)
  Enumerated Constant2/1 -> "NTC PASS "/3(NtcSts)
  Constant4/1 -> Relational Operator1/2
  Data Store Read1/1 -> MaxRawAvrg_HwNwtMtr/1, Relational Operator1/1
  Constant1/1 -> Max Raw Average Calculation/1(VEHSPDPTNUM1_ULS_U08)
  Constant5/1 -> Total Counter Updation/1(HWPTNUMSUB1_CNT_U08)

== system SF007A_SysFricLrng/SysFricLrng/SysFricLrngPer1/RunningAndCalibrationModes/FricLearning/CopyRight2 ==

== system SF007A_SysFricLrng/SysFricLrng/SysFricLrngPer1/RunningAndCalibrationModes/FricLearning/Gate Calculation ==
  SelHwAg : Inport
  IC : Inport  Port=2
  Add1 : Sum
  Constant2 : Constant  Value=HWPTNUMSUB1_CNT_U08
  Constant3 : Constant  Value=SysFricLrngFricHysHwAgPt
  Constant4 : Constant  OutDataTypeStr=uint8
      settings: AttributesFormatString=%<OutDataTypeStr>
  CopyRight2 : Subsystem  Description=|  mask(Copyright Information){none=on}
      | Copyright info block.                                               
      |                                                                     
      | Place copyright information at the top of every subsystem in design.
      mask prompts: none "No parameters"
      mask help: Place copyright information at the top of every subsystem in design.
      mask Display:
      | NxtrConf = 'Nexteer Confidential';
      | 
      | sys = bdroot; %handle for the current model ("system")
      | first = get_param(sys,'Created');
      | first = first(end-3:end);  %year is last four digits
      | 
      | last = get_param(sys,'LastModifiedDate');
      | if isempty(last)
      |     last = datestr(now,'yyyy');
      | else
      |     last = last(end-3:end);
      | end
      | 
      | if strcmp(first,last)
      |     fprintf('%s -- Copyright %s Nexteer',NxtrConf,first)
      | else
      |     fprintf('%s -- %s%s- %s Nexteer',NxtrConf,char(169),first,last)
      | end
  Logical Operator : Logic  AllPortsSameDT=off  OutDataTypeStr=boolean
  Logical Operator1 : Logic  Operator=OR  AllPortsSameDT=off  OutDataTypeStr=boolean
  Relational Operator : RelationalOperator  Operator=<  OutDataTypeStr=boolean
  Relational Operator1 : RelationalOperator  Operator=<  OutDataTypeStr=boolean
  Relational Operator2 : RelationalOperator  OutDataTypeStr=boolean
  Selector : Selector  IndexOptions=Index vector (port)  Indices=[1 3]  OutputSizes=1
  Selector1 : Selector  IndexOptions=Index vector (port)  Indices=[1 3]  OutputSizes=1
  While Iterator : WhileIterator  MaxIters=-1  ShowIterationPort=on
  Gate : Outport
  wires:
  IC/1 -> While Iterator/2
  Constant3/1 -> Selector/1, Selector1/1
  Constant2/1 -> Relational Operator/2
  Relational Operator/1 -> Logical Operator/1
  Add1/1 -> Selector1/2
  Constant4/1 -> Add1/2
  Logical Operator1/1 -> Logical Operator/2
  Logical Operator/1 -> While Iterator/1
  SelHwAg/1 -> [SelHwAg]
  [SelHwAg] -> Relational Operator1/1
  Selector/1 -> Relational Operator1/2
  Relational Operator1/1 -> Logical Operator1/1
  Selector1/1 -> Relational Operator2/2
  [SelHwAg] -> Relational Operator2/1
  Relational Operator2/1 -> Logical Operator1/2
  While Iterator/1 -> Gate/1, Relational Operator/1, Selector/2, Add1/1

== system SF007A_SysFricLrng/SysFricLrng/SysFricLrngPer1/RunningAndCalibrationModes/FricLearning/Indices Calculation ==
  note: Note: Model has one based Index logic for Indices calculation.
      | Code might use Zero based index. Mapping of values between
      | zero based and one based Index is given below
  note: Code: (Zero Based Index)                       ||   Model (One Based Index)
      | -----------------------------------------------------||----------------------------------------------------
      | VSIdx | OffsInc | OffsDec|Offs(0)|Offs(1) ||VSIdx | OffsInc | OffsDec|Offs(0)|Offs(1)
      | -----------------------------------------------------------------------------------------------------------
      |      0    |    0      |  1          |  0       |    1      ||   1      |   1         |  2         | 1      |   2
      |      1    |    2      |  3          |  2       |    3      ||   2      |   3         |  4         | 3      |   4
      |      2    |    4      |  5          |  4       |    5      ||   3      |   5         |  6         | 5      |   6
      |      3    |    6      |  7          |  6       |    7      ||   4      |   7         |  8         | 7      |   8
  note: Note: Mapping of values between Zero Based and one based Index
  HwVelDir : Inport
  VehSpdIdx : Inport  Port=2
  Add1 : Sum  Inputs=+-
  Add2 : Sum
  Add3 : Sum  Inputs=+-
  Constant1 : Constant  OutDataTypeStr=uint8
      settings: AttributesFormatString=%<OutDataTypeStr>
  Constant2 : Constant  Value=IDXCALCNSCAGFAC_ULS_U08
  Constant3 : Constant  OutDataTypeStr=uint8
      settings: AttributesFormatString=%<OutDataTypeStr>
  CopyRight2 : Subsystem  Description=|  mask(Copyright Information){none=on}
      | Copyright info block.                                               
      |                                                                     
      | Place copyright information at the top of every subsystem in design.
      mask prompts: none "No parameters"
      mask help: Place copyright information at the top of every subsystem in design.
      mask Display:
      | NxtrConf = 'Nexteer Confidential';
      | 
      | sys = bdroot; %handle for the current model ("system")
      | first = get_param(sys,'Created');
      | first = first(end-3:end);  %year is last four digits
      | 
      | last = get_param(sys,'LastModifiedDate');
      | if isempty(last)
      |     last = datestr(now,'yyyy');
      | else
      |     last = last(end-3:end);
      | end
      | 
      | if strcmp(first,last)
      |     fprintf('%s -- Copyright %s Nexteer',NxtrConf,first)
      | else
      |     fprintf('%s -- %s%s- %s Nexteer',NxtrConf,char(169),first,last)
      | end
  Product : Product
  DeltaIdxOffsInc : Outport
  DeltaIdxOffs : Outport  Port=2
  DeltaIdxOffsDec : Outport  Port=3
  wires:
  Product/1 -> DeltaIdxOffsDec/1, Add3/1, Add2/2
  HwVelDir/1 -> Add2/1
  Constant2/1 -> Product/2
  VehSpdIdx/1 -> Product/1
  Add3/1 -> DeltaIdxOffsInc/1
  Constant3/1 -> Add3/2
  Add2/1 -> Add1/1
  Add1/1 -> DeltaIdxOffs/1
  Constant1/1 -> Add1/2
